simulink model "Rail_CtlLoopParaMeUn"  (R2016b)
settings: configuration reference "CodeGenConfigSet" (kept outside this file)
values from neighbouring files (symbols this model uses):
  Rail_facMeUnCtlDCor_CUR = Calibration.Parameter    [init_Rail_CtlLoopParaMeUn.m]
  Rail_facMeUnCtlDCor_CURX = Calibration.Parameter    [init_Rail_CtlLoopParaMeUn.m]
  Rail_facMeUnCtlICor_CUR = Calibration.Parameter    [init_Rail_CtlLoopParaMeUn.m]
  Rail_facMeUnCtlICor_CURX = Calibration.Parameter    [init_Rail_CtlLoopParaMeUn.m]
  Rail_facMeUnCtlPCor_CUR = Calibration.Parameter    [init_Rail_CtlLoopParaMeUn.m]
  Rail_facMeUnCtlPCor_CURX = Calibration.Parameter    [init_Rail_CtlLoopParaMeUn.m]
  Rail_facMeUnCtlPT1_CUR = Calibration.Parameter    [init_Rail_CtlLoopParaMeUn.m]
  Rail_facMeUnCtlPT1_CURX = Calibration.Parameter    [init_Rail_CtlLoopParaMeUn.m]
  Rail_facOvrMeUnNegIncr_C = Calibration.Parameter    [init_Rail_CtlLoopParaMeUn.m]
  Rail_MeUnCtlDKd_CUR = Calibration.Parameter    [init_Rail_CtlLoopParaMeUn.m]
  Rail_MeUnCtlDKd_CURX = Calibration.Parameter    [init_Rail_CtlLoopParaMeUn.m]
  Rail_MeUnCtlIKi_CUR = Calibration.Parameter    [init_Rail_CtlLoopParaMeUn.m]
  Rail_MeUnCtlIKi_CURX = Calibration.Parameter    [init_Rail_CtlLoopParaMeUn.m]
  Rail_MeUnCtlIKiNeg_CUR = Calibration.Parameter    [init_Rail_CtlLoopParaMeUn.m]
  Rail_MeUnCtlIKiNeg_CURX = Calibration.Parameter    [init_Rail_CtlLoopParaMeUn.m]
  Rail_MeUnCtlIKiPos_CUR = Calibration.Parameter    [init_Rail_CtlLoopParaMeUn.m]
  Rail_MeUnCtlIKiPos_CURX = Calibration.Parameter    [init_Rail_CtlLoopParaMeUn.m]
  Rail_MeUnCtlPKp_CUR = Calibration.Parameter    [init_Rail_CtlLoopParaMeUn.m]
  Rail_MeUnCtlPKp_CURX = Calibration.Parameter    [init_Rail_CtlLoopParaMeUn.m]
  Rail_MeUnCtlPKpNeg_CUR = Calibration.Parameter    [init_Rail_CtlLoopParaMeUn.m]
  Rail_MeUnCtlPKpNeg_CURX = Calibration.Parameter    [init_Rail_CtlLoopParaMeUn.m]
  Rail_MeUnCtlPKpPos_CUR = Calibration.Parameter    [init_Rail_CtlLoopParaMeUn.m]
  Rail_MeUnCtlPKpPos_CURX = Calibration.Parameter    [init_Rail_CtlLoopParaMeUn.m]
  Rail_pOvrMeUnThresHigh_C = Calibration.Parameter    [init_Rail_CtlLoopParaMeUn.m]
  Rail_pOvrMeUnThresLow_C = Calibration.Parameter    [init_Rail_CtlLoopParaMeUn.m]
  Rail_tiMeUnCtlDT1_CUR = Calibration.Parameter    [init_Rail_CtlLoopParaMeUn.m]
  Rail_tiMeUnCtlDT1_CURX = Calibration.Parameter    [init_Rail_CtlLoopParaMeUn.m]
libraries: CXLib x1
settings Model: Creator=lenovo  LastModifiedBy=wangrui
settings ConfigSetRef: SourceLocation=Base Workspace

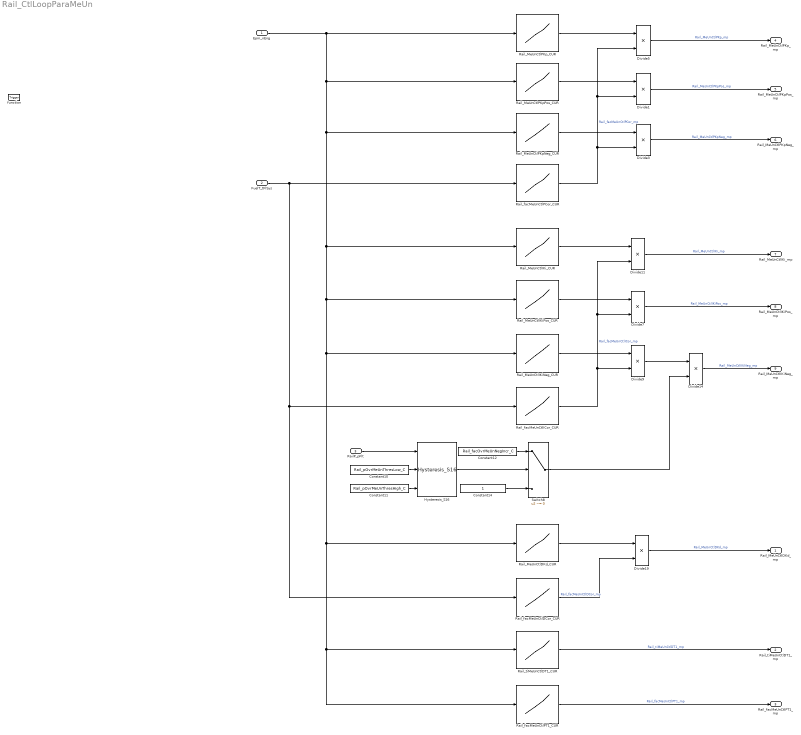
== system Rail_CtlLoopParaMeUn ==
  Epm_nEng : Inport  Tag=rpm  Description=Engine speed  OutMin=0  OutMax=6000  OutDataTypeStr=EngSpeed_rpm
  FuelT_tFlSys : Inport  Tag=deg  Description=Fuel system temperature  Port=2  OutMin=-50  OutMax=200  OutDataTypeStr=Temp_deg
  RailP_pFlt : Inport  Tag=bar  Description=Maximum rail pressure of the last 10 sampling cycle  Port=3  OutMin=0  OutMax=2500  OutDataTypeStr=RailPressure_bar
  function : TriggerPort  TriggerType=function-call  VariantControl=Variant
  Constant10 : Constant  Value=Rail_pOvrMeUnThresLow_C  SampleTime=-1
  Constant11 : Constant  Value=Rail_pOvrMeUnThresHigh_C  SampleTime=-1
  Constant12 : Constant  Value=Rail_facOvrMeUnNegIncr_C  SampleTime=-1
  Constant14 : Constant  OutDataTypeStr=Factor  SampleTime=-1
  Divide{1,3,5,7,9,11,14,19} (8 alike) : Product  Inputs=**  OutDataTypeStr=Inherit: Inherit via back propagation
  Hysteresis_S16 : CXLib/Hysteresis_S16
  Rail_MeUnCtlDKd_CUR : Lookup_n-D  NumberOfTableDimensions=1  BreakpointsForDimension1=Rail_MeUnCtlDKd_CURX  IndexSearchMethod=Linear search  BeginIndexSearchUsingPreviousIndexResult=on  Table=Rail_MeUnCtlDKd_CUR  ExtrapMethod=Clip  UseLastTableValue=on  InternalRulePriority=Speed  OutDataTypeStr=Inherit: Inherit via back propagation  SaturateOnIntegerOverflow=on
  Rail_MeUnCtlIKiNeg_CUR : Lookup_n-D  NumberOfTableDimensions=1  BreakpointsForDimension1=Rail_MeUnCtlIKiNeg_CURX  IndexSearchMethod=Linear search  BeginIndexSearchUsingPreviousIndexResult=on  Table=Rail_MeUnCtlIKiNeg_CUR  ExtrapMethod=Clip  UseLastTableValue=on  InternalRulePriority=Speed  OutDataTypeStr=Inherit: Inherit via back propagation  SaturateOnIntegerOverflow=on
  Rail_MeUnCtlIKiPos_CUR : Lookup_n-D  NumberOfTableDimensions=1  BreakpointsForDimension1=Rail_MeUnCtlIKiPos_CURX  IndexSearchMethod=Linear search  BeginIndexSearchUsingPreviousIndexResult=on  Table=Rail_MeUnCtlIKiPos_CUR  ExtrapMethod=Clip  UseLastTableValue=on  InternalRulePriority=Speed  OutDataTypeStr=Inherit: Inherit via back propagation  SaturateOnIntegerOverflow=on
  Rail_MeUnCtlIKi_CUR : Lookup_n-D  NumberOfTableDimensions=1  BreakpointsForDimension1=Rail_MeUnCtlIKi_CURX  IndexSearchMethod=Linear search  BeginIndexSearchUsingPreviousIndexResult=on  Table=Rail_MeUnCtlIKi_CUR  ExtrapMethod=Clip  UseLastTableValue=on  InternalRulePriority=Speed  OutDataTypeStr=Inherit: Inherit via back propagation  SaturateOnIntegerOverflow=on
  Rail_MeUnCtlPKpNeg_CUR : Lookup_n-D  NumberOfTableDimensions=1  BreakpointsForDimension1=Rail_MeUnCtlPKpNeg_CURX  IndexSearchMethod=Linear search  BeginIndexSearchUsingPreviousIndexResult=on  Table=Rail_MeUnCtlPKpNeg_CUR  ExtrapMethod=Clip  UseLastTableValue=on  InternalRulePriority=Speed  OutDataTypeStr=Inherit: Inherit via back propagation  SaturateOnIntegerOverflow=on
  Rail_MeUnCtlPKpPos_CUR : Lookup_n-D  NumberOfTableDimensions=1  BreakpointsForDimension1=Rail_MeUnCtlPKpPos_CURX  IndexSearchMethod=Linear search  BeginIndexSearchUsingPreviousIndexResult=on  Table=Rail_MeUnCtlPKpPos_CUR  ExtrapMethod=Clip  UseLastTableValue=on  InternalRulePriority=Speed  OutDataTypeStr=Inherit: Inherit via back propagation  SaturateOnIntegerOverflow=on
  Rail_MeUnCtlPKp_CUR : Lookup_n-D  NumberOfTableDimensions=1  BreakpointsForDimension1=Rail_MeUnCtlPKp_CURX  IndexSearchMethod=Linear search  BeginIndexSearchUsingPreviousIndexResult=on  Table=Rail_MeUnCtlPKp_CUR  ExtrapMethod=Clip  UseLastTableValue=on  InternalRulePriority=Speed  OutDataTypeStr=Inherit: Inherit via back propagation  SaturateOnIntegerOverflow=on
  Rail_facMeUnCtlDCor_CUR : Lookup_n-D  NumberOfTableDimensions=1  BreakpointsForDimension1=Rail_facMeUnCtlDCor_CURX  IndexSearchMethod=Linear search  BeginIndexSearchUsingPreviousIndexResult=on  Table=Rail_facMeUnCtlDCor_CUR  ExtrapMethod=Clip  UseLastTableValue=on  InternalRulePriority=Speed  OutDataTypeStr=Inherit: Inherit via back propagation  SaturateOnIntegerOverflow=on
  Rail_facMeUnCtlICor_CUR : Lookup_n-D  NumberOfTableDimensions=1  BreakpointsForDimension1=Rail_facMeUnCtlICor_CURX  IndexSearchMethod=Linear search  BeginIndexSearchUsingPreviousIndexResult=on  Table=Rail_facMeUnCtlICor_CUR  ExtrapMethod=Clip  UseLastTableValue=on  InternalRulePriority=Speed  OutDataTypeStr=Inherit: Inherit via back propagation  SaturateOnIntegerOverflow=on
  Rail_facMeUnCtlPCor_CUR : Lookup_n-D  NumberOfTableDimensions=1  BreakpointsForDimension1=Rail_facMeUnCtlPCor_CURX  IndexSearchMethod=Linear search  BeginIndexSearchUsingPreviousIndexResult=on  Table=Rail_facMeUnCtlPCor_CUR  ExtrapMethod=Clip  UseLastTableValue=on  InternalRulePriority=Speed  OutDataTypeStr=Inherit: Inherit via back propagation  SaturateOnIntegerOverflow=on
  Rail_facMeUnCtlPT1_CUR : Lookup_n-D  NumberOfTableDimensions=1  BreakpointsForDimension1=Rail_facMeUnCtlPT1_CURX  IndexSearchMethod=Linear search  BeginIndexSearchUsingPreviousIndexResult=on  Table=Rail_facMeUnCtlPT1_CUR  ExtrapMethod=Clip  UseLastTableValue=on  InternalRulePriority=Speed  OutDataTypeStr=Inherit: Inherit via back propagation  SaturateOnIntegerOverflow=on
  Rail_tiMeUnCtlDT1_CUR : Lookup_n-D  NumberOfTableDimensions=1  BreakpointsForDimension1=Rail_tiMeUnCtlDT1_CURX  IndexSearchMethod=Linear search  BeginIndexSearchUsingPreviousIndexResult=on  Table=Rail_tiMeUnCtlDT1_CUR  ExtrapMethod=Clip  UseLastTableValue=on  InternalRulePriority=Speed  OutDataTypeStr=Inherit: Inherit via back propagation  SaturateOnIntegerOverflow=on
  Switch8 : Switch  Criteria=u2 ~= 0  InputSameDT=on
  Rail_MeUnCtlDKd_mp : Outport  Description=D amplification for pressure control by metering unit  OutMin=0  OutMax=15  OutDataTypeStr=Pid_Kp_Kd
  Rail_tiMeUnCtlDT1_mp : Outport  Tag=ms  Description=Time constant of the DT1 element for pressure control by metering unit  Port=2  OutMin=0  OutMax=65535  OutDataTypeStr=RailDT1_ms
  Rail_facMeUnCtlPT1_mp : Outport  Description=Time constant of the PT1 filter for pressure control by metering unit  Port=3  OutMin=0  OutMax=99.9985  OutDataTypeStr=PT_fac
  Rail_MeUnCtlPKp_mp : Outport  Description=P-Gain within the window  Port=4  OutMin=0  OutMax=15  OutDataTypeStr=Pid_Kp_Kd
  Rail_MeUnCtlPKpPos_mp : Outport  Description=P-gain above upper window border  Port=5  OutMin=0  OutMax=15  OutDataTypeStr=Pid_Kp_Kd
  Rail_MeUnCtlPKpNeg_mp : Outport  Description=P-gain below lower window border  Port=6  OutMin=0  OutMax=15  OutDataTypeStr=Pid_Kp_Kd
  Rail_MeUnCtlIKi_mp : Outport  Description=I-Gain within the window  Port=7  OutMin=0  OutMax=65  OutDataTypeStr=Pid_Ki
  Rail_MeUnCtlIKiPos_mp : Outport  Description=I-Gain above upper window border  Port=8  OutMin=0  OutMax=65  OutDataTypeStr=Pid_Ki
  Rail_MeUnCtlIKiNeg_mp : Outport  Description=I-Gain below upper window border  Port=9  OutMin=0  OutMax=65  OutDataTypeStr=Pid_Ki
  wires:
  Divide3/1 -> Rail_MeUnCtlPKpNeg_mp/1  "Rail_MeUnCtlPKpNeg_mp"
  Divide1/1 -> Rail_MeUnCtlPKpPos_mp/1  "Rail_MeUnCtlPKpPos_mp"
  Rail_MeUnCtlPKp_CUR/1 -> Divide5/1
  Divide14/1 -> Rail_MeUnCtlIKiNeg_mp/1  "Rail_MeUnCtlIKiNeg_mp"
  Rail_facMeUnCtlPCor_CUR/1 -> Divide3/2, Divide1/2, Divide5/2  "Rail_facMeUnCtlPCor_mp"
  Rail_MeUnCtlPKpPos_CUR/1 -> Divide1/1
  Constant10/1 -> Hysteresis_S16/2
  Rail_MeUnCtlPKpNeg_CUR/1 -> Divide3/1
  Divide11/1 -> Rail_MeUnCtlIKi_mp/1  "Rail_MeUnCtlIKi_mp"
  Divide5/1 -> Rail_MeUnCtlPKp_mp/1  "Rail_MeUnCtlPKp_mp"
  FuelT_tFlSys/1 -> Rail_facMeUnCtlDCor_CUR/1, Rail_facMeUnCtlICor_CUR/1, Rail_facMeUnCtlPCor_CUR/1
  Rail_MeUnCtlIKi_CUR/1 -> Divide11/1
  Divide7/1 -> Rail_MeUnCtlIKiPos_mp/1  "Rail_MeUnCtlIKiPos_mp"
  Rail_MeUnCtlIKiPos_CUR/1 -> Divide7/1
  Rail_MeUnCtlIKiNeg_CUR/1 -> Divide9/1
  Rail_facMeUnCtlICor_CUR/1 -> Divide9/2, Divide7/2, Divide11/2  "Rail_facMeUnCtlICor_mp"
  Constant12/1 -> Switch8/1
  RailP_pFlt/1 -> Hysteresis_S16/1
  Constant11/1 -> Hysteresis_S16/3
  Divide9/1 -> Divide14/1
  Hysteresis_S16/1 -> Switch8/2
  Rail_facMeUnCtlPT1_CUR/1 -> Rail_facMeUnCtlPT1_mp/1  "Rail_facMeUnCtlPT1_mp"
  Rail_tiMeUnCtlDT1_CUR/1 -> Rail_tiMeUnCtlDT1_mp/1  "Rail_tiMeUnCtlDT1_mp"
  Switch8/1 -> Divide14/2
  Constant14/1 -> Switch8/3
  Divide19/1 -> Rail_MeUnCtlDKd_mp/1  "Rail_MeUnCtlDKd_mp"
  Rail_facMeUnCtlDCor_CUR/1 -> Divide19/2  "Rail_facMeUnCtlDCor_mp"
  Rail_MeUnCtlDKd_CUR/1 -> Divide19/1
  Epm_nEng/1 -> Rail_MeUnCtlPKp_CUR/1, Rail_MeUnCtlPKpPos_CUR/1, Rail_MeUnCtlDKd_CUR/1, Rail_tiMeUnCtlDT1_CUR/1, Rail_facMeUnCtlPT1_CUR/1, Rail_MeUnCtlIKiNeg_CUR/1, Rail_MeUnCtlIKiPos_CUR/1, Rail_MeUnCtlIKi_CUR/1, Rail_MeUnCtlPKpNeg_CUR/1
